simulink model "PMSM_Simulation_2025a"  (R2025a)
settings: Solver=FixedStepDiscrete  StartTime=0.0  StopTime=10.0  FixedStep=0.0000625/200  RelTol=1e-3
values from neighbouring files (symbols this model uses):
  MC_DCurrLopKi_CFG = 0.009    [PMSM_MC_Data_2025a.sldd]
  MC_DCurrLopKp_CFG = 2.763    [PMSM_MC_Data_2025a.sldd]
  MC_MotModeDebug_CFG = 5.0    [PMSM_MC_Data_2025a.sldd]
  MC_POLE_NUM_CFG = 4.0    [PMSM_MC_Data_2025a.sldd]
  MC_QCurrLopKi_CFG = 0.009    [PMSM_MC_Data_2025a.sldd]
  MC_QCurrLopKp_CFG = 2.763    [PMSM_MC_Data_2025a.sldd]
  MC_SpdLopKi_CFG = 0.0001    [PMSM_MC_Data_2025a.sldd]
  MC_SpdLopKp_CFG = 0.006    [PMSM_MC_Data_2025a.sldd]
libraries: simulink x16, slpidlib x3, spsDCVoltageSourceLib x1, spsPermanentMagnetSynchronousMachineLib x1, spsUniversalBridgeLib x1, sps_lib x1
(part 2 of 2)

== system PMSM_Simulation_2025a/PMSM_MC/MC_HighFrqTask/FOC/SVPWM/SevenSegSVPWM/SectorCaculate ==
  Ualpha : Inport
  Ubeta : Inport  Port=2
  A : Fcn  Expr=u[2]
  Add : Sum  Inputs=+++
  B : Fcn  Expr=u(1)*sqrt(3/4)-0.5*u[2]
  C : Fcn  Expr=-u[1]*sqrt(3/4)-u[2]*0.5
  Constant : Constant  Value=uint8(1)
  Constant1 : Constant  Value=uint8(0)
  Data Type Conversion : DataTypeConversion  OutDataTypeStr=uint8  SaturateOnIntegerOverflow=off  RndMeth=Floor
  Gain : Gain  Gain=2
  Gain1 : Gain  Gain=4
  Mux : Mux  Inputs=2
  Switch : Switch  Criteria=u2 > Threshold  SaturateOnIntegerOverflow=off  InputSameDT=off
  Switch1 : Switch  Criteria=u2 > Threshold  SaturateOnIntegerOverflow=off  InputSameDT=off
  Switch2 : Switch  Criteria=u2 > Threshold  SaturateOnIntegerOverflow=off  InputSameDT=off
  N : Outport
  wires:
  Ualpha/1 -> Mux/1
  Ubeta/1 -> Mux/2
  Mux/1 -> C/1, A/1, B/1
  A/1 -> Switch/2
  B/1 -> Switch1/2
  C/1 -> Switch2/2
  Constant/1 -> Switch/1, Switch2/1, Switch1/1
  Constant1/1 -> Switch/3, Switch1/3, Switch2/3
  Switch2/1 -> Gain1/1
  Switch1/1 -> Gain/1
  Gain/1 -> Add/2
  Gain1/1 -> Add/3
  Switch/1 -> Add/1
  Add/1 -> Data Type Conversion/1
  Data Type Conversion/1 -> N/1

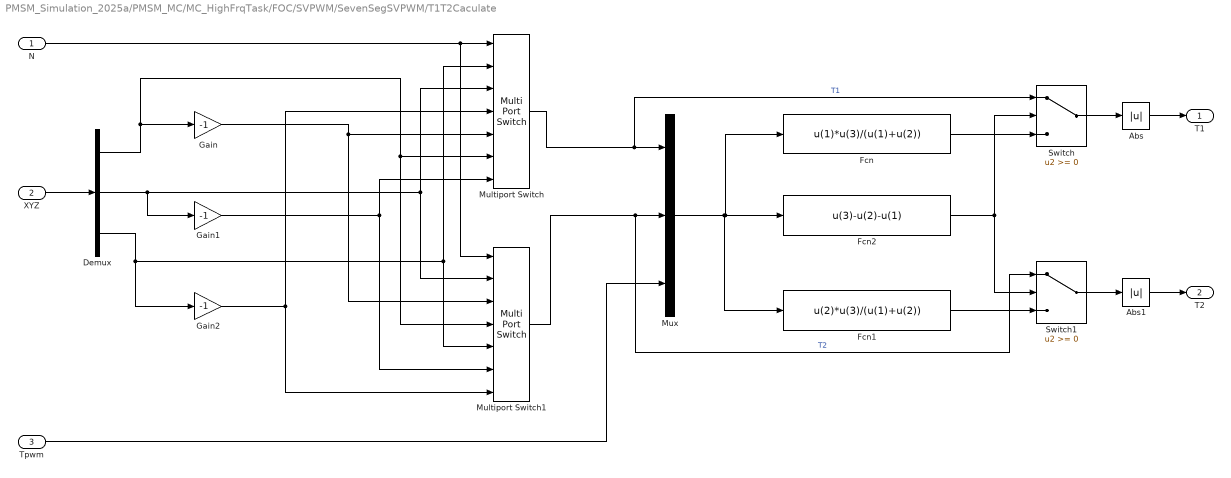
== system PMSM_Simulation_2025a/PMSM_MC/MC_HighFrqTask/FOC/SVPWM/SevenSegSVPWM/T1T2Caculate ==
  N : Inport
  XYZ : Inport  Port=2
  Tpwm : Inport  Port=3
  Abs : Abs  SaturateOnIntegerOverflow=off
  Abs1 : Abs  SaturateOnIntegerOverflow=off
  Demux : Demux  Outputs=3
  Fcn : Fcn  Expr=u(1)*u(3)/(u(1)+u(2))
  Fcn1 : Fcn  Expr=u(2)*u(3)/(u(1)+u(2))
  Fcn2 : Fcn  Expr=u(3)-u(2)-u(1)
  Gain : Gain  Gain=-1
  Gain1 : Gain  Gain=-1
  Gain2 : Gain  Gain=-1
  Multiport Switch : MultiPortSwitch  Inputs=6  DiagnosticForDefault=None  SaturateOnIntegerOverflow=off  InputSameDT=off
  Multiport Switch1 : MultiPortSwitch  Inputs=6  DiagnosticForDefault=None  SaturateOnIntegerOverflow=off  InputSameDT=off
  Mux : Mux  Inputs=3
  Switch : Switch  SaturateOnIntegerOverflow=off  InputSameDT=off
  Switch1 : Switch  SaturateOnIntegerOverflow=off  InputSameDT=off
  T1 : Outport
  T2 : Outport  Port=2
  wires:
  N/1 -> Multiport Switch/1, Multiport Switch1/1
  XYZ/1 -> Demux/1
  Demux/1 -> Gain/1, Multiport Switch/6, Multiport Switch1/4
  Demux/2 -> Gain1/1, Multiport Switch/3, Multiport Switch1/2
  Demux/3 -> Gain2/1, Multiport Switch1/5, Multiport Switch/2
  Gain/1 -> Multiport Switch1/3, Multiport Switch/5
  Gain2/1 -> Multiport Switch1/7, Multiport Switch/4
  Gain1/1 -> Multiport Switch/7, Multiport Switch1/6
  Multiport Switch/1 -> Switch/1, Mux/1  "T1"
  Multiport Switch1/1 -> Switch1/1, Mux/2  "T2"
  Tpwm/1 -> Mux/3
  Mux/1 -> Fcn1/1, Fcn/1, Fcn2/1
  Fcn/1 -> Switch/3
  Fcn1/1 -> Switch1/3
  Fcn2/1 -> Switch1/2, Switch/2
  Switch/1 -> Abs/1
  Abs/1 -> T1/1
  Switch1/1 -> Abs1/1
  Abs1/1 -> T2/1

== system PMSM_Simulation_2025a/PMSM_MC/MC_HighFrqTask/FOC/SVPWM/SevenSegSVPWM/TcmCaculate ==
  N : Inport
  T1 : Inport  Port=2
  T2 : Inport  Port=3
  Tpwm : Inport  Port=4
  Fcn : Fcn  Expr=(u(3)+u(1)+u(2))/2
  Fcn1 : Fcn  Expr=(u(3)-u(1)+u(2))/2
  Fcn2 : Fcn  Expr=(u(3)-u(1)-u(2))/2
  Multiport Switch : MultiPortSwitch  Inputs=6  DiagnosticForDefault=None  SaturateOnIntegerOverflow=off  InputSameDT=off
  Multiport Switch1 : MultiPortSwitch  Inputs=6  DiagnosticForDefault=None  SaturateOnIntegerOverflow=off  InputSameDT=off
  Multiport Switch2 : MultiPortSwitch  Inputs=6  DiagnosticForDefault=None  SaturateOnIntegerOverflow=off  InputSameDT=off
  Mux : Mux  Inputs=3
  Mux1 : Mux  Inputs=3
  Tcm1 Tcm2 Tcm3 : Outport
  wires:
  Mux/1 -> Tcm1 Tcm2 Tcm3/1
  T2/1 -> Mux1/2
  T1/1 -> Mux1/1
  Tpwm/1 -> Mux1/3
  Mux1/1 -> Fcn/1, Fcn2/1, Fcn1/1
  N/1 -> Multiport Switch2/1, Multiport Switch1/1, Multiport Switch/1
  Fcn1/1 -> Multiport Switch1/4, Multiport Switch/7, Multiport Switch/2, Multiport Switch1/5, Multiport Switch2/6, Multiport Switch2/3
  Fcn/1 -> Multiport Switch1/6, Multiport Switch2/7, Multiport Switch2/5, Multiport Switch/4, Multiport Switch/3, Multiport Switch1/2
  Fcn2/1 -> Multiport Switch1/7, Multiport Switch/6, Multiport Switch/5, Multiport Switch1/3, Multiport Switch2/4, Multiport Switch2/2
  Multiport Switch/1 -> Mux/1
  Multiport Switch1/1 -> Mux/2
  Multiport Switch2/1 -> Mux/3

== system PMSM_Simulation_2025a/PMSM_MC/MC_HighFrqTask/FOC/SVPWM/SevenSegSVPWM/XYZCaculate ==
  Ualpha : Inport
  Ubeta : Inport  Port=2
  Udc : Inport  Port=3
  Ts : Inport  Port=4
  Add : Sum
  Add1 : Sum  Inputs=+-
  Fcn : Fcn  Expr=1/u
  Gain : Gain  Gain=3/2
  Gain1 : Gain  Gain=sqrt(3)
  Gain2 : Gain  Gain=sqrt(3)/2
  Mux : Mux  Inputs=3
  Product{,1..3} (4 alike) : Product
  XYZ : Outport
  wires:
  Ualpha/1 -> Gain/1
  Ubeta/1 -> Gain2/1, Gain1/1
  Gain/1 -> Add/2, Add1/2
  Gain1/1 -> Product/1
  Gain2/1 -> Add1/1, Add/1
  Ts/1 -> Product3/1
  Product3/1 -> Product1/2, Product/2, Product2/2
  Add/1 -> Product1/1
  Udc/1 -> Fcn/1
  Fcn/1 -> Product3/2
  Add1/1 -> Product2/1
  Product1/1 -> Mux/2
  Product2/1 -> Mux/3
  Product/1 -> Mux/1
  Mux/1 -> XYZ/1

== stateflow chart PMSM_Simulation_2025a/PMSM_MC/MC_HighFrqTask/OpenLopMod/OpenLopThetaeCal ==
  state Stop
    en:
    //init output
    Thetae_SensLess = 0;
    OLStartCompletedFlag = 0;
    //init local variable
    WeRefRamped = 0;
  state VFOpenLoop
    state Align
      en:
      Thetae_SensLess = 0;
    state Open
      en,du:
      Ramping(OLWeRef,OLWeRampMaxStep);
      OLThetaeSum();
      Thetae_SensLess = Thetae_OL;
    (default) -> VFOpenLoop.Align
    VFOpenLoop.Align -> VFOpenLoop.Open : [after(100,msec)]
  state IFStart
    state Align
      en:
      Thetae_SensLess = 0;
    state Open
      en,du:
      Ramping(OLWeRef,OLWeRampMaxStep);
      OLThetaeSum();
      Thetae_SensLess = Thetae_OL;
    (default) -> IFStart.Align
    IFStart.Align -> IFStart.Open : [after(100,msec)]
  state Ramping(in,MaxStep) [function]
    note: WeRefRamped指当前的局部真实被电机使用的一个设定速度值，电机最开始为0，当我的速度期望值比较大的时候，就会与现在的WeRefRamped真实速度设定值比较，让他以MaxStep的递增速度累加或者累减，直到设定值与期望值的差值在[-MaxStep,+MaxStep]时，将当前速度赋值给定成期望值
    (default) -> (junction 23)
    (junction 23) -> (junction 30) [order 1] : [in - WeRefRamped > MaxStep]
    (junction 23) -> (junction 32) [order 2]
    (junction 30) -> (junction 41) : {
        | WeRefRamped = WeRefRamped + MaxStep;
        | }
    (junction 32) -> (junction 34) [order 1] : [in - WeRefRamped < -MaxStep]
    (junction 32) -> (junction 36) [order 2] : {
        | WeRefRamped = in;
        | }
    (junction 34) -> (junction 38) : {
        | WeRefRamped = WeRefRamped - MaxStep;
        | }
    (junction 38) -> (junction 36)
    (junction 41) -> (junction 38)
    (junction 36) -> (junction 43)
  state OLThetaeSum [function]
    note: MotCtrMode==8条件是为了VF开环使用的，
        | 我们的VF开环只进行正向累加，而MotorSpdRef
        | 主要用于IF启动的时候使用
    (default) -> (junction 28)
    (junction 28) -> (junction 48) [order 1] : [MotorSpdRef > 0||...
        | MotCtrMode == 8]
    (junction 28) -> (junction 52) [order 2] : {
        | Thetae_OL = Thetae_OL - WeRefRamped*Ts;
        | }
    (junction 48) -> (junction 50) : {
        | Thetae_OL = Thetae_OL + WeRefRamped*Ts;
        | }
    (junction 50) -> (junction 52)
    (junction 52) -> (junction 55)
    (junction 55) -> (junction 57) [order 1] : [Thetae_OL < 0]
    (junction 55) -> (junction 59) [order 2] : {
        | //set range to [0 2pi]
        | Thetae_OL = fmod(Thetae_OL,6.28);
        | }
    (junction 57) -> (junction 58) : {
        | //set range to [0 2pi]
        | Thetae_OL  = -Thetae_OL;
        | Thetae_OL = fmod(Thetae_OL,6.28);
        | Thetae_OL =  6.28 - Thetae_OL;
        | }
    (junction 58) -> (junction 59)
    (junction 59) -> (junction 60)
  (default) -> Stop
  Stop -> VFOpenLoop [order 1] : [MotCtrMode==8]
  VFOpenLoop -> Stop : [MotCtrMode!=8]
  Stop -> IFStart [order 2] : [MotCtrMode==7]
  data: in function_input double; MaxStep function_input double; MotCtrMode input uint8; Wm_Est input single; Thetae_Est input single; MotorSpdRef input int16; OLWeRef input single; OLWeRampMaxStep input single; OLSpdStableThd input single; OLSpdStableCnt input single; Ts input single; Thetae_SensLess output single; OLStartCompletedFlag output boolean; WeRefRamped local single; OLWeightedTransmTime input single; Thetae_OL local single

== stateflow chart PMSM_Simulation_2025a/Scheduler ==
  (default) -> (junction 6)
  (junction 6) -> (junction 11) [order 1] : [counter%%3200==3199]
  (junction 6) -> (junction 10) [order 2]
  (junction 11) -> (junction 9) : {trig_MidFrq_1ms;}
  (junction 9) -> (junction 10)
  (junction 10) -> (junction 36)
  (junction 36) -> (junction 38) [order 1] : [counter%%200==199]
  (junction 36) -> (junction 41) [order 2]
  (junction 38) -> (junction 40) : {trig_HighFrq_62_5us;}
  (junction 40) -> (junction 41)
  (junction 41) -> (junction 18)
  (junction 18) -> (junction 20) [order 1] : [counter>=100000000]
  (junction 18) -> (junction 24) [order 2] : {counter++;}
  (junction 20) -> (junction 22) : {counter=0;}
  (junction 22) -> (junction 24)
  (junction 24) -> (junction 27)
  data: counter local uint32 =0
  events: trig_MidFrq_1ms output FUNCTION_CALL_EVENT; trig_HighFrq_62_5us output FUNCTION_CALL_EVENT

== stateflow chart PMSM_Simulation_2025a/PMSM_MC/MC_LowFrqTask/MotModeCtr/ModeMgr ==
  state RangeCheck [function]
    (default) -> (junction 21)
    (junction 21) -> (junction 23) [order 1] : [abs(MotOffsetBuff[0]-MotOffsetBuff[1])>100]
    (junction 21) -> (junction 24) [order 2] : {
        | MotCalNormal=1;
        | MotOffset = (MotOffsetBuff[0]+MotOffsetBuff[1])/2;
        | }
    (junction 23) -> (junction 25) : {MotCalNormal=0;}
    (junction 25) -> (junction 24)
    (junction 24) -> (junction 35)
  state SensorCtr
    state Calibrate
      state Init
        en:
        MotCtrMode=0;
      state Calibrate1
        en:
        MotCtrMode=1;
        MotCalThetae = 1.046;//60°
      state Calibrate2
        en:
        MotOffsetBuff[0]=Ecode_cnt-166;
        MotCtrMode=2;
        MotCalThetae = 2.093;//120°
      state RngChk
        en:
        MotOffsetBuff[1]=Ecode_cnt-333;
        RangeCheck();
      (default) -> Init
      Init -> Calibrate1 : [MotorSpdRef != 0]
      Calibrate1 -> Calibrate2 : [after(1.5,sec)]
      Calibrate2 -> RngChk : [after(1.5,sec)]
    state Normal
      state Stop
        en:
        MotCtrMode=4;
      state Run
        en:
        MotCtrMode=5;
      (default) -> SensorCtr.Normal.Stop
      SensorCtr.Normal.Run -> SensorCtr.Normal.Stop : [MotorSpdRef==0]
      SensorCtr.Normal.Stop -> SensorCtr.Normal.Run : [MotorSpdRef!=0]
    state CalFailed
      en:
      MotCtrMode=3;
    (default) -> Calibrate
    CalFailed -> Calibrate : [MotorSpdRef==0]
    RngChk -> CalFailed [order 1] : [MotCalNormal==0]
    RngChk -> Normal [order 2] : [MotCalNormal==1]
  state SensorLessCtr
    state Stop
      en:
      MotCtrMode=4;
    state StartFail
      en:
      MotCtrMode=6;
    state IFStart
      en:
      MotCtrMode=7;
    state Run
      en:
      MotCtrMode=5;
    (default) -> SensorLessCtr.Stop
    SensorLessCtr.Stop -> IFStart : [MotorSpdRef != 0]
    StartFail -> SensorLessCtr.Stop : [MotorSpdRef==0]
    SensorLessCtr.Run -> SensorLessCtr.Stop : [MotorSpdRef==0]
    IFStart -> StartFail [order 2] : [after(600,msec)]
    IFStart -> SensorLessCtr.Run [order 1] : [OLStartCompletedFlag==1]
  note: 注意此处的无感有感开环状态机
      | 的切换模式条件中，如果是仿真
      | 测试需要把速度设定改成不等于
      | 0，但是嵌入式模型部署中需要
      | 改成等于0
  state VFOpenLoop
    en:
    MotCtrMode = 8;
  (default) -> SensorCtr
  SensorCtr -> SensorLessCtr [order 1] : [//value is 1 mean sensorless control
      | SensorLessEn ==1 &&...
      | MotorSpdRef != 0]
  SensorLessCtr -> SensorCtr [order 1] : [//value is 0 mean sensor control
      | SensorLessEn ==0 &&...
      | MotorSpdRef != 0]
  SensorLessCtr -> VFOpenLoop [order 2] : [OpenLoopEn == 1&&...
      | MotorSpdRef != 0]
  VFOpenLoop -> SensorLessCtr [order 1] : [OpenLoopEn == 0&&...
      | MotorSpdRef != 0&&...
      | SensorLessEn == 1]
  VFOpenLoop -> SensorCtr [order 2] : [OpenLoopEn == 0&&...
      | MotorSpdRef != 0&&...
      | SensorLessEn == 0]
  SensorCtr -> VFOpenLoop [order 2] : [OpenLoopEn == 1&&...
      | MotorSpdRef != 0]
  data: MotCtrMode output uint8; Ecode_cnt input int32; MotorSpdRef input int16; MotOffset output int32; MotCalThetae output single; MotOffsetBuff local int32 size=2; MotCalNormal local boolean; SensorLessEn input boolean; OpenLoopEn input boolean; OLStartCompletedFlag input boolean
